simulink model "consigna_posicion_entrada"  (R2023b)
settings: Solver=VariableStepAuto  StartTime=0.0  StopTime=15  RelTol=1e-3
libraries: simulink x3
settings Model: Creator=rodri  LastModifiedBy=Nahuel

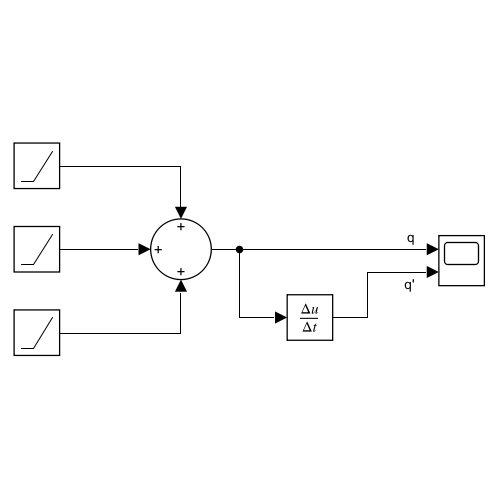
[thumbnail: Simulink's stored preview of the top-level diagram]
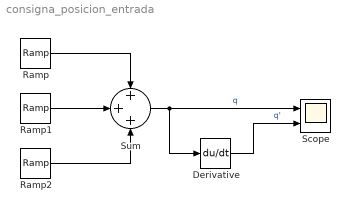
== system consigna_posicion_entrada ==
  Derivative : Derivative
  Ramp : simulink/Sources/Ramp  slope=2*pi/5  start=0  InitialOutput=0
  Ramp1 : simulink/Sources/Ramp  slope=-2*pi/5  start=5  InitialOutput=0
  Ramp2 : simulink/Sources/Ramp  slope=-2*pi/5  start=10  InitialOutput=0
  Scope : Scope  NumInputPorts=2
  Sum : Sum  Inputs=+++
  wires:
  Ramp/1 -> Sum/1
  Ramp1/1 -> Sum/2
  Sum/1 -> Derivative/1, Scope/1  "q"
  Ramp2/1 -> Sum/3
  Derivative/1 -> Scope/2  "q'"
